simulink library "hcu_lib"  (R2021b)
settings: Solver=VariableStepAuto  StartTime=0.0  StopTime=10.0  RelTol=1e-3
undefined symbols (not defined in the file): ENUM_FAULTSTATE_FAIL, ENUM_FAULTSTATE_INDETERMINATE, ENUM_FAULTSTATE_PASS, EPSILON, FALSE, KPH2MPH, KPH2MPS, KXX2XX, MPH2KPH, MPS2KPH, ONE_INT, ONE_INT16, ONE_INT32, RADPS2RPM, RPM2RADPS, slcm, TRUE, UNDEFINED_VALUE, XX2KXX, ZERO_FLOAT, ZERO_INT, ZERO_INT16, ZERO_INT32
libraries: $bdroot x29, simulink x12, afl x1
(part 2 of 3)

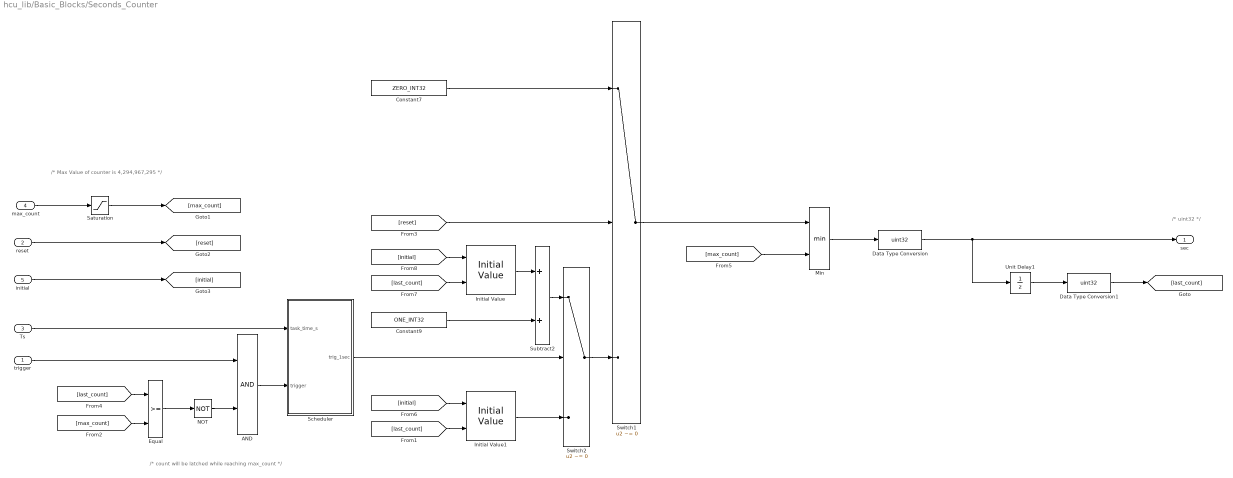
== system hcu_lib/Basic_Blocks/Seconds_Counter ==
  note: /* count will be latched while reaching max_count */
  note: /* uint32 */
  note: /* Max Value of counter is 4,294,967,295 */
  trigger : Inport
  reset : Inport  Port=2
  Ts : Inport  Port=3
  max_count : Inport  Port=4
  initial : Inport  Port=5
  AND : Logic  AllPortsSameDT=off  OutDataTypeStr=boolean
  Constant7 : Constant  Value=ZERO_INT32  OutDataTypeStr=uint16
  Constant9 : Constant  Value=ONE_INT32  OutDataTypeStr=single
  Data Type Conversion : DataTypeConversion  OutDataTypeStr=uint32
  Data Type Conversion1 : DataTypeConversion  OutDataTypeStr=uint32
  Equal : RelationalOperator  OutDataTypeStr=boolean  RndMeth=Simplest
  Initial Value : $bdroot/Basic_Blocks/Initial Value
  Initial Value1 : $bdroot/Basic_Blocks/Initial Value
  Min : MinMax  Inputs=2
  NOT : Logic  Operator=NOT  AllPortsSameDT=off  OutDataTypeStr=boolean
  Saturation : Saturate  UpperLimit=4294967295  LowerLimit=0
      settings: AttributesFormatString=<upper = %<UpperLimit>>\n<lower = %<LowerLimit>>
  Scheduler : Stateflow chart  TreatAsAtomicUnit=on
  Subtract2 : Sum
  Switch1 : Switch  Criteria=u2 ~= 0
      settings: AttributesFormatString=<%<Criteria>>
  Switch2 : Switch  Criteria=u2 ~= 0
      settings: AttributesFormatString=<%<Criteria>>
  Unit Delay1 : UnitDelay  SampleTime=-1  HasFrameUpgradeWarning=on
      settings: AttributesFormatString=<initial = %<X0>>
  sec : Outport
  wires:
  Data Type Conversion1/1 -> [last_count]
  Unit Delay1/1 -> Data Type Conversion1/1
  Data Type Conversion/1 -> Unit Delay1/1, sec/1
  Ts/1 -> Scheduler/1(task_time_s)
  Subtract2/1 -> Switch2/1
  Constant9/1 -> Subtract2/2
  Switch2/1 -> Switch1/3
  Constant7/1 -> Switch1/1
  max_count/1 -> Saturation/1
  Scheduler/1(trig_1sec) -> Switch2/2
  reset/1 -> [reset]
  [reset] -> Switch1/2
  Equal/1 -> NOT/1
  AND/1 -> Scheduler/2(trigger)
  trigger/1 -> AND/1
  NOT/1 -> AND/2
  [last_count] -> Equal/1
  Saturation/1 -> [max_count]
  [max_count] -> Equal/2
  [max_count] -> Min/2
  Min/1 -> Data Type Conversion/1
  Switch1/1 -> Min/1
  initial/1 -> [initial]
  Initial Value1/1 -> Switch2/3
  [last_count] -> Initial Value1/2
  [initial] -> Initial Value1/1
  Initial Value/1 -> Subtract2/1
  [initial] -> Initial Value/1
  [last_count] -> Initial Value/2

== system hcu_lib/Basic_Blocks/Test Detection Criteria ==
  trigger : Inport
  Ts : Inport  Port=2
  KDDM_xxxDTC_cnt : Inport  Port=3
  KDDM_xxxDetTO_s : Inport  Port=4
  Constant35 : Constant  Value=ZERO_INT
  Data Type Conversion : DataTypeConversion  OutDataTypeStr=single
  Data Type Conversion1 : DataTypeConversion  OutDataTypeStr=uint16
  Detect Increase : simulink/Logic and Bit Operations/Detect Increase  vinit=0.0  OutDataTypeStr=boolean
  Equal9 : RelationalOperator  Operator===  OutDataTypeStr=boolean  RndMeth=Simplest
  Gain : Gain  Gain=KXX2XX  RndMeth=Round
  Gain1 : Gain  Gain=KXX2XX
  Logical Operator19 : Logic  AllPortsSameDT=off  OutDataTypeStr=boolean
  Logical Operator3 : Logic  Operator=NOT  AllPortsSameDT=off  OutDataTypeStr=boolean
  ModMath : Subsystem  mask(Count){}
      mask help: Counter function.
      mask Display:
      | fprintf('ModMath');
      | port_label('output', 1, 'Remainder');
      | port_label('input', 1, 'Dividend');
      | port_label('input', 2, 'Divisor');
  Product : Product
  Rounding Function : Rounding  Operator=round
  Rounding Function1 : Rounding  Operator=round
  Timer : Subsystem  mask(Timer){}
      mask help: Timer funcion.
  VDDM_xxxDet_flg : Outport
  wires:
  Constant35/1 -> Equal9/2
  Logical Operator19/1 -> Detect Increase/1
  trigger/1 -> Timer/1(trigger), Logical Operator19/1, Logical Operator3/1
  [KDDM_xxxDetTO_s] -> Gain1/1
  Equal9/1 -> Logical Operator19/2
  Logical Operator3/1 -> Timer/2(reset)
  Timer/1(time) -> Gain/1
  Ts/1 -> Timer/3(Ts)
  Product/1 -> Timer/4(max_time)
  Data Type Conversion/1 -> Product/2
  KDDM_xxxDetTO_s/1 -> [KDDM_xxxDetTO_s], Product/1
  KDDM_xxxDTC_cnt/1 -> Data Type Conversion/1
  ModMath/1(Remainder) -> Data Type Conversion1/1
  Detect Increase/1 -> VDDM_xxxDet_flg/1
  Gain/1 -> Rounding Function/1
  Gain1/1 -> Rounding Function1/1
  Data Type Conversion1/1 -> Equal9/1
  Rounding Function/1 -> ModMath/1(Dividend)
  Rounding Function1/1 -> ModMath/2(Divisor)

== system hcu_lib/Basic_Blocks/Timer ==
  note: /* output signal type is single */
  trigger : Inport
  reset : Inport  Port=2
  Ts : Inport  Port=3
  max_time : Inport  Port=4
  Constant1 : Constant  Value=ZERO_FLOAT  OutDataTypeStr=single
  GreaterThan : RelationalOperator  Operator=<=  OutDataTypeStr=boolean  RndMeth=Simplest
  Subtract2 : Sum
  Switch : Switch  Criteria=u2 > Threshold
  Switch1 : Switch  Criteria=u2 ~= 0
      settings: AttributesFormatString=<%<Criteria>>
  Switch2 : Switch  Criteria=u2 ~= 0
      settings: AttributesFormatString=<%<Criteria>>
  Unit Delay1 : UnitDelay  SampleTime=-1  HasFrameUpgradeWarning=on
      settings: AttributesFormatString=<initial = %<X0>>
  time : Outport
  wires:
  [last_time] -> Subtract2/1
  max_time/1 -> Switch/1, GreaterThan/1
  Unit Delay1/1 -> [last_time], Switch1/3
  Switch/1 -> time/1, Unit Delay1/1
  Switch2/1 -> Switch/3, GreaterThan/2
  Ts/1 -> Subtract2/2
  Switch1/1 -> Switch2/3
  Constant1/1 -> Switch1/1
  reset/1 -> Switch1/2
  trigger/1 -> Switch2/2
  Subtract2/1 -> Switch2/1
  GreaterThan/1 -> Switch/2

== system hcu_lib/Basic_Blocks/derivative ==
  omega_radps : Inport
  task_time_s : Inport  Port=2
  Constant : Constant  Tag=struct('comment',struct('text','','placement',1),'output',struct('width',1,'name','$S_$B','unit','','type','Int16','offset',0,'max',NaN,'min',NaN,'freeze',1,'lsb',1,'arb',0,'class','default','address','','description','','value','0','tolerance',1,'show',0),'date',731450.689904282)  Value=0  OutDataTypeStr=single
  Constant1 : Constant  Tag=struct('comment',struct('text','','placement',1),'output',struct('width',1,'name','$S_$B','unit','','type','Int16','offset',0,'max',NaN,'min',NaN,'freeze',1,'lsb',1,'arb',0,'class','default','address','','description','','value','2','tolerance',1,'show',0),'date',731450.690075)  Value=TRUE
  Product : Product  Tag=struct('comment',struct('text','','placement',1),'logdata',struct('maxnumvals',inf,'plotchannels',[],'stepsize',0,'downsampling',1,'loggingmode',3,'channels',1),'output',struct('width',1,'name','$S_$B','unit','','type','Int32Bin15','offset',0,'max',65535,'min',-65536,'freeze',1,'lsb',2^-15,'arb',0,'class','default','address','','description','','autoscalingmode',1,'lowerheadroom',1,'upperheadroom',1,'headroomunit','bit','checkmin',0,'checkmax',0,'show',0),'inputs','*/','exceptionhandling',1,'date',731458.438505301)  Inputs=*/  InputSameDT=on  RndMeth=Zero  SaturateOnIntegerOverflow=on  OutDataTypeStr=Inherit: Same as first input
  Saturation1 : Saturate  Tag=struct('comment',struct('text','','placement',1),'logdata',struct('maxnumvals',inf,'plotchannels',[],'stepsize',0,'downsampling',1,'loggingmode',3,'channels',1),'output',struct('width',1,'name','$S_$B','unit','s','type','Time16bin10','offset',0,'max',63.999,'min',0,'freeze',1,'lsb',2^-10,'arb',0,'class','default','address','','description','','autoscalingmode',1,'lowerheadroom',1,'upperheadroom',1,'headroomunit','bit','show',0),'lowerlimit',struct('width',1,'name','$S_$B_lower','unit','','type','Int16','offset',0,'max',NaN,'min',NaN,'freeze',1,'lsb',1,'arb',0,'class','default','address','','description','','value','12e-3','scalar',0),'upperlimit',struct('width',1,'name','$S_$B_upper','unit','','type','Int16','offset',0,'max',NaN,'min',NaN,'freeze',1,'lsb',1,'arb',0,'class','default','address','','description','','value','63.9','scalar',0),'date',731458.439118333)  UpperLimit=63.9  LowerLimit=12e-3
  Saturation2 : Saturate  Tag=struct('comment',struct('text','','placement',1),'logdata',struct('maxnumvals',inf,'plotchannels',[],'stepsize',0,'downsampling',1,'loggingmode',3,'channels',1),'output',struct('width',1,'name','$S_$B','unit','','type','Int32Bin15','offset',0,'max',65535,'min',-65536,'freeze',1,'lsb',2^-15,'arb',0,'class','default','address','','description','','autoscalingmode',1,'lowerheadroom',1,'upperheadroom',1,'headroomunit','bit','show',0),'lowerlimit',struct('width',1,'name','$S_$B_lower','unit','','type','Int16','offset',0,'max',NaN,'min',NaN,'freeze',1,'lsb',1,'arb',0,'class','default','address','','description','','value','-65536','scalar',0),'upperlimit',struct('width',1,'name','$S_$B_upper','unit','','type','Int16','offset',0,'max',NaN,'min',NaN,'freeze',1,'lsb',1,'arb',0,'class','default','address','','description','','value','65535','scalar',0),'date',731455.58891853)  UpperLimit=65535  LowerLimit=-65536
  Sum : Sum  Tag=struct('comment',struct('text','','placement',1),'logdata',struct('maxnumvals',inf,'plotchannels',[],'stepsize',0,'downsampling',1,'loggingmode',3,'channels',1),'output',struct('width',1,'name','$S_$B','unit','','type','Int32Bin15','offset',0,'max',65535,'min',-65536,'freeze',1,'lsb',2^-15,'arb',0,'class','default','address','','description','','autoscalingmode',1,'lowerheadroom',1,'upperheadroom',1,'headroomunit','bit','checkmin',0,'checkmax',0,'show',0),'inputs','+-','date',731450.688943275)  Inputs=+-  InputSameDT=on  SaturateOnIntegerOverflow=on  OutDataTypeStr=Inherit: Same as first input
  Switch : Switch  Tag=struct('comment',struct('text','','placement',1),'logdata',struct('maxnumvals',inf,'plotchannels',[],'stepsize',0,'downsampling',1,'loggingmode',3,'channels',1),'output',struct('width',1,'name','$S_$B','unit','','type','Int32Bin15','offset',0,'max',65535,'min',-65536,'freeze',1,'lsb',2^-15,'arb',0,'class','default','address','','description','','autoscalingmode',1,'lowerheadroom',1,'upperheadroom',1,'headroomunit','bit','checkmin',0,'checkmax',0,'show',0),'threshold',struct('width',1,'name','$S_$B_threshold','unit','','type','Int16','offset',0,'max',NaN,'min',NaN,'freeze',1,'lsb',1,'arb',0,'class','default','address','','description','','value','1','scalar',0),'date',731458.438569977)  Threshold=0.5  SaturateOnIntegerOverflow=on  InputSameDT=on
  UnitDelay1 : UnitDelay  Tag=struct('comment',struct('text','','placement',1),'logdata',struct('maxnumvals',inf,'plotchannels',[],'stepsize',0,'downsampling',1,'loggingmode',3,'channels',1),'output',struct('width',1,'name','$S_$B','unit','','type','Int32Bin15','offset',0,'max',65535,'min',-65536,'freeze',1,'lsb',2^-15,'arb',0,'class','default','address','','description','','autoscalingmode',1,'lowerheadroom',1,'upperheadroom',1,'headroomunit','bit','checkmin',0,'checkmax',0,'show',0,'initial','0'),'state',0,'dt','-1','date',731450.687911019)  SampleTime=-1  HasFrameUpgradeWarning=on
  UnitDelay2 : UnitDelay  Tag=struct('comment',struct('text','','placement',1),'logdata',struct('maxnumvals',inf,'plotchannels',[],'stepsize',0,'downsampling',1,'loggingmode',3,'channels',1),'output',struct('width',1,'name','$S_$B','unit','','type','UInt8','offset',0,'max',255,'min',0,'freeze',1,'lsb',1,'arb',0,'class','default','address','','description','','autoscalingmode',1,'lowerheadroom',1,'upperheadroom',1,'headroomunit','bit','checkmin',0,'checkmax',0,'show',0,'initial','0'),'state',0,'dt','-1','date',731450.690382801)  InitialCondition=FALSE  SampleTime=-1  StateName=first_pass  HasFrameUpgradeWarning=on
  rot_acc_radps2 : Outport
  wires:
  Saturation1/1 -> Product/2
  Constant1/1 -> UnitDelay2/1
  UnitDelay2/1 -> Switch/2
  Constant/1 -> Switch/3  "zero"
  Switch/1 -> Product/1
  task_time_s/1 -> Saturation1/1
  Sum/1 -> Switch/1
  Product/1 -> Saturation2/1
  UnitDelay1/1 -> Sum/2
  Saturation2/1 -> rot_acc_radps2/1  "rot_acc_radps2"
  omega_radps/1 -> Sum/1, UnitDelay1/1

== system hcu_lib/Basic_Blocks/divide ==
  dividend : Inport
  divisor : Inport  Port=2
  default_value : Inport  Port=3
  Divide : Product  Inputs=*/
  Interval Test : simulink/Logic and Bit Operations/Interval Test  IntervalClosedRight=on  uplimit=single(0.00001)  IntervalClosedLeft=on  lowlimit=single(-0.00001)  OutDataTypeStr=boolean
  Logical Operator : Logic  Operator=NOT  Inputs=1  AllPortsSameDT=off  OutDataTypeStr=boolean
  Switch : Switch  Threshold=0.5
  quotient : Outport
  wires:
  Logical Operator/1 -> Switch/2
  default_value/1 -> Switch/3  "default_value"
  Interval Test/1 -> Logical Operator/1
  Switch/1 -> quotient/1
  Divide/1 -> Switch/1
  divisor/1 -> Interval Test/1, Divide/2  "divisor"
  dividend/1 -> Divide/1  "dividend"

== system hcu_lib/Basic_Blocks/rolling average ==
  note: new_average = [ (sample_interval)/(sample_interval + time_constant) ] * (new_value - old_ave) + old_ave
  note: - (FK_TMR/TC)
      |                                    f  =  1  -  e
      |
      |       Where "f" is called the filter constant in the difference equation:
      |
      |                    new_average = f * new_value + (1 - f) * old_average
  note: Using the first two terms of the series expansion:
      |
      |                     x                     x2
      |                                e   =  1  +  x  +  --  + ......
      |                                           2!
      |
      |       Simplifying, the exponential "f" becomes:
      |
      |                  - (FK_TMR/TC)              1
      |           f  =  1  -  e                    =  1  -  -------------  =  . . .
      |                                                    (FK_TMR/TC)
      |                           e
      |
      |                              1                      1
      |          f  =  1  -  ---------------------------------  =    ------------------- .
      |                                  1 + (FK_TMR / TC)       1 + (TC / FK_TMR)
  new_value : Inport
  old_ave : Inport  Port=2
  delta_t : Inport  Port=3
  tc : Inport  Port=4
  IC : UnitDelay  Tag=struct('comment',struct('text','','placement',1),'logdata',struct('maxnumvals',inf,'plotchannels',[],'stepsize',0,'downsampling',1,'loggingmode',3,'channels',1),'output',struct('width',1,'name','$S_$B','unit','','type','Int16','offset',0,'max',NaN,'min',NaN,'freeze',1,'lsb',1,'arb',0,'class','default','address','','description','','autoscalingmode',1,'lowerheadroom',1,'upperheadroom',1,'headroomunit','bit','checkmin',0,'checkmax',0,'show',0,'initial','2'),'state',0,'dt','-1','date',731455.586925799)  InitialCondition=1  SampleTime=-1  HasFrameUpgradeWarning=on
  Product_tmp1 : Product  Tag=struct('comment',struct('text','','placement',1),'logdata',struct('maxnumvals',inf,'plotchannels',[],'stepsize',0,'downsampling',1,'loggingmode',3,'channels',1),'output',struct('width',1,'name','$S_$B','unit','','type','Int32Bin15','offset',0,'max',65535,'min',-65536,'freeze',1,'lsb',2^-15,'arb',0,'class','default','address','','description','','autoscalingmode',1,'lowerheadroom',1,'upperheadroom',1,'headroomunit','bit','checkmin',0,'checkmax',0,'show',0),'inputs','**','exceptionhandling',1,'date',731455.58640515)  Inputs=**  InputSameDT=on  RndMeth=Zero  OutDataTypeStr=Inherit: Same as first input
  Sum : Sum  Tag=struct('comment',struct('text','','placement',1),'logdata',struct('maxnumvals',inf,'plotchannels',[],'stepsize',0,'downsampling',1,'loggingmode',3,'channels',1),'output',struct('width',1,'name','$S_$B','unit','','type','Int32Bin15','offset',0,'max',65535,'min',-65536,'freeze',1,'lsb',2^-15,'arb',0,'class','default','address','','description','','autoscalingmode',1,'lowerheadroom',1,'upperheadroom',1,'headroomunit','bit','checkmin',0,'checkmax',0,'show',0),'inputs','-+','date',731455.586330463)  Inputs=-+  InputSameDT=on  OutDataTypeStr=Inherit: Same as first input
  Sum1 : Sum  Tag=struct('comment',struct('text','','placement',1),'logdata',struct('maxnumvals',inf,'plotchannels',[],'stepsize',0,'downsampling',1,'loggingmode',3,'channels',1),'output',struct('width',1,'name','$S_$B','unit','','type','Int32Bin15','offset',0,'max',65535,'min',-65536,'freeze',1,'lsb',2^-15,'arb',0,'class','default','address','','description','','autoscalingmode',1,'lowerheadroom',1,'upperheadroom',1,'headroomunit','bit','checkmin',0,'checkmax',0,'show',0),'inputs','++','date',731455.58628235)  InputSameDT=on  OutDataTypeStr=Inherit: Same as first input
  Sum2 : Sum  Tag=struct('comment',struct('text','','placement',1),'logdata',struct('maxnumvals',inf,'plotchannels',[],'stepsize',0,'downsampling',1,'loggingmode',3,'channels',1),'output',struct('width',1,'name','$S_$B','unit','','type','Int32Bin15','offset',0,'max',65535,'min',-65536,'freeze',1,'lsb',2^-15,'arb',0,'class','default','address','','description','','autoscalingmode',1,'lowerheadroom',1,'upperheadroom',1,'headroomunit','bit','checkmin',0,'checkmax',0,'show',0),'inputs','++','date',731455.586506424)  InputSameDT=on  OutDataTypeStr=Inherit: Same as first input
  Switch1 : Switch  Tag=struct('comment',struct('text','','placement',1),'logdata',struct('maxnumvals',inf,'plotchannels',[],'stepsize',0,'downsampling',1,'loggingmode',3,'channels',1),'output',struct('width',1,'name','$S_$B','unit','','type','Int32Bin15','offset',0,'max',65535,'min',-65536,'freeze',1,'lsb',2^-15,'arb',0,'class','default','address','','description','','autoscalingmode',1,'lowerheadroom',1,'upperheadroom',1,'headroomunit','bit','checkmin',0,'checkmax',0,'show',0),'threshold',struct('width',1,'name','$S_$B_threshold','unit','','type','Int16','offset',0,'max',NaN,'min',NaN,'freeze',1,'lsb',1,'arb',0,'class','default','address','','description','','value','1','scalar',0),'date',731455.58657044)  Threshold=0.5  InputSameDT=on
  divide : $bdroot/Basic_Blocks/divide
  zero : Constant  Tag=struct('comment',struct('text','','placement',1),'output',struct('width',1,'name','$S_$B','unit','','type','Int16','offset',0,'max',NaN,'min',NaN,'freeze',1,'lsb',1,'arb',0,'class','default','address','','description','','value','0','tolerance',1,'show',0),'date',731455.58675544)  Value=0  OutDataTypeStr=Inherit: Inherit via back propagation
  zero1 : Constant  Tag=struct('comment',struct('text','','placement',1),'output',struct('width',1,'name','$S_$B','unit','','type','Int16','offset',0,'max',NaN,'min',NaN,'freeze',1,'lsb',1,'arb',0,'class','default','address','','description','','value','0','tolerance',1,'show',0),'date',731455.58675544)  Value=0  OutDataTypeStr=Inherit: Inherit via back propagation
  new_ave : Outport
  wires:
  zero1/1 -> divide/3
  Product_tmp1/1 -> divide/1
  [new_value] -> Switch1/1
  Switch1/1 -> new_ave/1  "new_ave"
  Sum2/1 -> Switch1/3  "new_ave"
  IC/1 -> Switch1/2
  zero/1 -> IC/1
  Sum1/1 -> divide/2
  Sum/1 -> Product_tmp1/1
  divide/1 -> Sum2/2
  tc/1 -> Sum1/2
  delta_t/1 -> Sum1/1, Product_tmp1/2  "delta_t"
  new_value/1 -> [new_value]  "new_value"
  old_ave/1 -> Sum2/1, Sum/1  "old_ave"
  [new_value] -> Sum/2

== system hcu_lib/IO_Signal_Process_Blocks/CAN_Msg_Validity_Process ==
  signal_in : Inport
  inverse_flag : Inport  Port=2
  debounce_sat : Inport  Port=3
  debounce_inc : Inport  Port=4
  debounce_dec : Inport  Port=5
  cal_override_flag : Inport  Port=6
  cal_override_value : Inport  Port=7
  service_flag : Inport  Port=8
  service_value : Inport  Port=9
  AFL : afl/AFL  SystemSampleTime=-1
  Ground : Ground
  Ground1 : Ground
  Ground2 : Ground
  Logical Operator : Logic  Operator=NOT  Inputs=1  AllPortsSameDT=off  OutDataTypeStr=boolean
  SRS_HCU_INP_003 : simulink/Model-Wide Utilities/DocBlock  DocumentType=Text
  Switch1 : Switch  Criteria=u2 ~= 0  Threshold=0.5
  Terminator : Terminator
  Terminator1 : Terminator
  Terminator2 : Terminator
  "override_signal_m2 " : $bdroot/Signal_Process_Blocks/override_signal_m2 
  signal_out : Outport  OutDataTypeStr=boolean
  wires:
  "override_signal_m2 "/1 -> signal_out/1
  AFL/3 -> Terminator/1
  "override_signal_m2 "/2 -> Terminator1/1
  AFL/1 -> "override_signal_m2 "/2
  Ground/1 -> "override_signal_m2 "/1
  service_flag/1 -> "override_signal_m2 "/3
  service_value/1 -> "override_signal_m2 "/4
  cal_override_flag/1 -> "override_signal_m2 "/5
  cal_override_value/1 -> "override_signal_m2 "/6
  inverse_flag/1 -> Switch1/2
  signal_in/1 -> Switch1/3, Logical Operator/1
  Switch1/1 -> AFL/1
  Logical Operator/1 -> Switch1/1
  AFL/2 -> Terminator2/1
  debounce_sat/1 -> AFL/2
  debounce_inc/1 -> AFL/3
  debounce_dec/1 -> AFL/4
  Ground1/1 -> AFL/5
  Ground2/1 -> AFL/6

== system hcu_lib/IO_Signal_Process_Blocks/Protect ==
  in : Inport
  Bias : Bias  Bias=1
  Bitwise Operator : simulink/Logic and Bit Operations/Bitwise Operator  logicop=NOT  UseBitMask=off  BitMask=bin2dec('11011001')  BitMaskRealWorld=Stored Integer
  out : Outport
  wires:
  Bitwise Operator/1 -> Bias/1
  Bias/1 -> out/1
  in/1 -> Bitwise Operator/1

== system hcu_lib/IO_Signal_Process_Blocks/RollCnt ==
  max : Inport
  Add : Sum
  Constant : Constant  OutDataTypeStr=Inherit: Inherit via back propagation
  Constant1 : Constant  Value=0  OutDataTypeStr=Inherit: Inherit via back propagation
  Data Type Conversion6 : DataTypeConversion  OutDataTypeStr=uint8
  Relational Operator : RelationalOperator  Operator=>  OutDataTypeStr=boolean  RndMeth=Nearest
  Switch2 : Switch  Criteria=u2 ~= 0
  Unit Delay1 : UnitDelay  SampleTime=-1  HasFrameUpgradeWarning=on
      settings: AttributesFormatString=<initial=%<X0>>
  out : Outport
  wires:
  Constant/1 -> Add/1
  Add/1 -> Switch2/3, Relational Operator/1
  Unit Delay1/1 -> Add/2
  Constant1/1 -> Switch2/1
  Switch2/1 -> Unit Delay1/1, Data Type Conversion6/1
  max/1 -> Relational Operator/2
  Relational Operator/1 -> Switch2/2
  Data Type Conversion6/1 -> out/1

== system hcu_lib/IO_Signal_Process_Blocks/RollCntValid ==
  RollCnt : Inport
  TimeOut : Inport  Port=2
  Ts : Inport  Port=3
  Add : Sum
  RESET : Constant  Value=0  OutDataTypeStr=single
  Relational Operator1 : RelationalOperator  Operator===  OutDataTypeStr=boolean  RndMeth=Nearest
  Relational Operator2 : RelationalOperator  Operator=<  OutDataTypeStr=boolean  RndMeth=Nearest
  Switch : Switch  Criteria=u2 ~= 0
  Unit Delay : UnitDelay  SampleTime=-1  HasFrameUpgradeWarning=on
  Unit Delay1 : UnitDelay  SampleTime=-1  HasFrameUpgradeWarning=on
  valid : Outport
  wires:
  Ts/1 -> Add/2
  Add/1 -> Switch/1
  Unit Delay/1 -> Add/1
  RollCnt/1 -> Unit Delay1/1, Relational Operator1/2
  Unit Delay1/1 -> Relational Operator1/1
  Switch/1 -> Unit Delay/1, Relational Operator2/1
  Relational Operator1/1 -> Switch/2
  RESET/1 -> Switch/3
  TimeOut/1 -> Relational Operator2/2
  Relational Operator2/1 -> valid/1

== system hcu_lib/IO_Signal_Process_Blocks/can_signal_process ==
  signal_in : Inport
  signal_valid_in : Inport  Port=2
  msg_valid : Inport  Port=3
  default_value : Inport  Port=4
  fault_filter_lim : Inport  Port=5
  fault_filter_inc : Inport  Port=6
  fault_filter_dec : Inport  Port=7
  invalid_override : Inport  Port=8
  valid_override : Inport  Port=9
  cal_ovrdflg : Inport  Port=10
  cal_ovrdval : Inport  Port=11
  service_flag : Inport  Port=12
  service_value : Inport  Port=13
  Logical Operator1 : Logic  Operator=NOT  AllPortsSameDT=off  OutDataTypeStr=boolean
  Logical Operator2 : Logic  AllPortsSameDT=off  OutDataTypeStr=boolean
  "override_signal_m2 " : $bdroot/Signal_Process_Blocks/override_signal_m2 
  sig_valid_check : $bdroot/Signal_Process_Blocks/sig_valid_check
  signal_out : Outport
  signal_valid_out : Outport  Port=2
  wires:
  "override_signal_m2 "/2 -> signal_valid_out/1
  "override_signal_m2 "/1 -> signal_out/1
  msg_valid/1 -> Logical Operator2/2
  signal_in/1 -> sig_valid_check/1
  signal_valid_in/1 -> Logical Operator2/1
  Logical Operator2/1 -> sig_valid_check/2
  invalid_override/1 -> sig_valid_check/3
  Logical Operator1/1 -> "override_signal_m2 "/1  "signal_valid_flg_raw"
  service_flag/1 -> "override_signal_m2 "/3
  service_value/1 -> "override_signal_m2 "/4
  cal_ovrdflg/1 -> "override_signal_m2 "/5
  cal_ovrdval/1 -> "override_signal_m2 "/6
  valid_override/1 -> sig_valid_check/4
  default_value/1 -> sig_valid_check/5
  fault_filter_lim/1 -> sig_valid_check/6
  fault_filter_inc/1 -> sig_valid_check/7
  fault_filter_dec/1 -> sig_valid_check/8
  sig_valid_check/1 -> Logical Operator1/1  "fault_flg"
  sig_valid_check/2 -> "override_signal_m2 "/2  "valid_flg"

== system hcu_lib/IO_Signal_Process_Blocks/digital_signal_process ==
  signal_in : Inport
  inverse_flag : Inport  Port=2
  debounce_sat : Inport  Port=3
  debounce_inc : Inport  Port=4
  debounce_dec : Inport  Port=5
  cal_override_flag : Inport  Port=6
  cal_override_value : Inport  Port=7
  service_flag : Inport  Port=8
  service_value : Inport  Port=9
  Ground : Ground
  Logical Operator : Logic  Operator=NOT  Inputs=1  AllPortsSameDT=off  OutDataTypeStr=boolean
  Switch1 : Switch  Criteria=u2 ~= 0  Threshold=0.5
  Terminator : Terminator
  Terminator1 : Terminator
  fault_filter_reset : Subsystem  AncestorBlock=hcu_lib/Signal_Process_Blocks/fault_filter_reset  TreatAsAtomicUnit=on  RTWFcnName=ff_reset  RTWFileName=HCU_LIB  mask(FaultFilterReset){}
      mask help: Fault filter reset.
      settings: RTWFcnNameOpts=Use subsystem name  RTWFileNameOpts=User specified
  "override_signal_m2 " : $bdroot/Signal_Process_Blocks/override_signal_m2 
  signal_out : Outport  OutDataTypeStr=boolean
  wires:
  debounce_dec/1 -> fault_filter_reset/4(dec)
  debounce_inc/1 -> fault_filter_reset/3(inc)
  debounce_sat/1 -> fault_filter_reset/2(sat)
  "override_signal_m2 "/1 -> signal_out/1
  fault_filter_reset/2(ff_count) -> Terminator/1
  "override_signal_m2 "/2 -> Terminator1/1
  fault_filter_reset/1(fault_flg) -> "override_signal_m2 "/2
  Ground/1 -> "override_signal_m2 "/1
  service_flag/1 -> "override_signal_m2 "/3
  service_value/1 -> "override_signal_m2 "/4
  cal_override_flag/1 -> "override_signal_m2 "/5
  cal_override_value/1 -> "override_signal_m2 "/6
  inverse_flag/1 -> Switch1/2
  signal_in/1 -> Switch1/3, Logical Operator/1
  Switch1/1 -> fault_filter_reset/1(i_deb)
  Logical Operator/1 -> Switch1/1

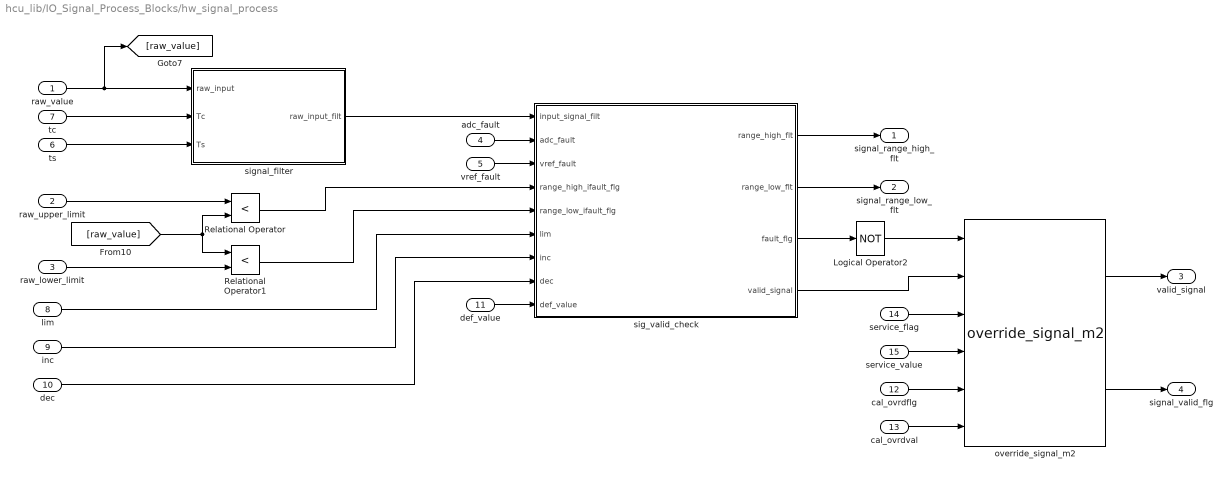
== system hcu_lib/IO_Signal_Process_Blocks/hw_signal_process ==
  raw_value : Inport
  raw_upper_limit : Inport  Port=2
  raw_lower_limit : Inport  Port=3
  adc_fault : Inport  Port=4
  vref_fault : Inport  Port=5
  ts : Inport  Port=6
  tc : Inport  Port=7
  lim : Inport  Port=8
  inc : Inport  Port=9
  dec : Inport  Port=10
  def_value : Inport  Port=11
  cal_ovrdflg : Inport  Port=12
  cal_ovrdval : Inport  Port=13
  service_flag : Inport  Port=14
  service_value : Inport  Port=15
  Logical Operator2 : Logic  Operator=NOT  AllPortsSameDT=off  OutDataTypeStr=boolean
  Relational Operator : RelationalOperator  Operator=<  OutDataTypeStr=boolean  RndMeth=Nearest
  Relational Operator1 : RelationalOperator  Operator=<  OutDataTypeStr=boolean  RndMeth=Nearest
  "override_signal_m2 " : $bdroot/Signal_Process_Blocks/override_signal_m2 
  sig_valid_check : Subsystem  RTWFcnName=sig_valid_check
      settings: RTWFcnNameOpts=User specified
  signal_filter : Subsystem
  signal_range_high_flt : Outport
  signal_range_low_flt : Outport  Port=2
  valid_signal : Outport  Port=3
  signal_valid_flg : Outport  Port=4
  wires:
  Logical Operator2/1 -> "override_signal_m2 "/1
  ts/1 -> signal_filter/3(Ts)
  tc/1 -> signal_filter/2(Tc)
  raw_value/1 -> [raw_value], signal_filter/1(raw_input)
  Relational Operator/1 -> sig_valid_check/4(range_high_ifault_flg)
  [raw_value] -> Relational Operator1/1, Relational Operator/2
  def_value/1 -> sig_valid_check/9(def_value)
  dec/1 -> sig_valid_check/8(dec)
  inc/1 -> sig_valid_check/7(inc)
  lim/1 -> sig_valid_check/6(lim)
  raw_lower_limit/1 -> Relational Operator1/2
  raw_upper_limit/1 -> Relational Operator/1
  sig_valid_check/3(fault_flg) -> Logical Operator2/1
  signal_filter/1(raw_input_filt) -> sig_valid_check/1(input_signal_filt)
  Relational Operator1/1 -> sig_valid_check/5(range_low_ifault_flg)
  sig_valid_check/1(range_high_flt) -> signal_range_high_flt/1
  sig_valid_check/2(range_low_flt) -> signal_range_low_flt/1
  service_flag/1 -> "override_signal_m2 "/3
  service_value/1 -> "override_signal_m2 "/4
  cal_ovrdflg/1 -> "override_signal_m2 "/5
  cal_ovrdval/1 -> "override_signal_m2 "/6
  sig_valid_check/4(valid_signal) -> "override_signal_m2 "/2
  "override_signal_m2 "/1 -> valid_signal/1
  "override_signal_m2 "/2 -> signal_valid_flg/1
  adc_fault/1 -> sig_valid_check/2(adc_fault)
  vref_fault/1 -> sig_valid_check/3(vref_fault)

== system hcu_lib/IO_Signal_Process_Blocks/signal_out ==
  in : Inport
  srvcflg : Inport  Port=2
  srvcval : Inport  Port=3
  ovrdflg : Inport  Port=4
  ovrdval : Inport  Port=5
  Constant1 : Constant  Value=TRUE  OutDataTypeStr=Inherit: Inherit via back propagation
  Terminator13 : Terminator
  "override_signal_m2 " : $bdroot/Signal_Process_Blocks/override_signal_m2 
  out : Outport
  wires:
  in/1 -> "override_signal_m2 "/2
  "override_signal_m2 "/1 -> out/1
  Constant1/1 -> "override_signal_m2 "/1
  srvcflg/1 -> "override_signal_m2 "/3
  srvcval/1 -> "override_signal_m2 "/4
  ovrdflg/1 -> "override_signal_m2 "/5
  ovrdval/1 -> "override_signal_m2 "/6
  "override_signal_m2 "/2 -> Terminator13/1

== system hcu_lib/Model Info1/EmptySubsystem ==

== system hcu_lib/Signal_Conversion_Blocks/Raw32 ==
  input : Inport
  gain : Inport  Port=2
  offset : Inport  Port=3
  Add1 : Sum  Inputs=+-
  Constant : Constant  Value=EPSILON
  Data Type Conversion6 : DataTypeConversion  OutDataTypeStr=uint32
  Divide : Product  Inputs=*/
  MinMax : MinMax  Function=max  Inputs=2
  Rounding Function : Rounding  Operator=round
  raw_value : Outport
  wires:
  Data Type Conversion6/1 -> raw_value/1
  Rounding Function/1 -> Data Type Conversion6/1
  input/1 -> Add1/1
  offset/1 -> Add1/2
  Add1/1 -> Divide/1
  Divide/1 -> Rounding Function/1
  gain/1 -> MinMax/1
  MinMax/1 -> Divide/2
  Constant/1 -> MinMax/2

== system hcu_lib/Signal_Conversion_Blocks/conv_counts_to_eng_units ==
  signal : Inport
  gain : Inport  Port=2
  offset : Inport  Port=3
  Product : Product  RndMeth=Zero
  Sum : Sum
  output_signal : Outport
  wires:
  Product/1 -> Sum/1
  gain/1 -> Product/1  "gain"
  signal/1 -> Product/2  "signal"
  offset/1 -> Sum/2  "offset"
  Sum/1 -> output_signal/1  "output_signal"

== system hcu_lib/Signal_Conversion_Blocks/conv_eng_units_to_counts ==
  input : Inport
  gain : Inport  Port=2
  offset : Inport  Port=3
  Constant : Constant  Value=0  OutDataTypeStr=Inherit: Inherit via back propagation
  Sum : Sum  Inputs=+-
  divide : $bdroot/Basic_Blocks/divide
  output_signal : Outport
  wires:
  Constant/1 -> divide/3
  offset/1 -> Sum/2  "offset"
  input/1 -> Sum/1  "input"
  gain/1 -> divide/2  "gain"
  Sum/1 -> divide/1  "out_signal"
  divide/1 -> output_signal/1  "output_signal"

== system hcu_lib/Signal_Conversion_Blocks/convert_in ==
  raw32 : Inport
  Add : Sum
  Data Type Conversion : DataTypeConversion  OutDataTypeStr=single
  Product : Product  RndMeth=Zero
  gain : Constant  Value=single(gain)  OutDataTypeStr=single
  offset : Constant  Value=single(offset)  OutDataTypeStr=single
  value : Outport
  wires:
  raw32/1 -> Data Type Conversion/1
  gain/1 -> Product/2
  Product/1 -> Add/1
  offset/1 -> Add/2
  Add/1 -> value/1
  Data Type Conversion/1 -> Product/1

== system hcu_lib/Signal_Conversion_Blocks/convert_out ==
  value : Inport
  Add : Sum  Inputs=+-
  Constant : Constant  Value=EPSILON
  Data Type Conversion : DataTypeConversion  OutDataTypeStr=uint32  RndMeth=Nearest
  Divide : Product  Inputs=*/
  MinMax : MinMax  Function=max  Inputs=2
  gain : Constant  Value=single(gain)  OutDataTypeStr=single
  offset : Constant  Value=single(offset)  OutDataTypeStr=single
  raw32 : Outport
  wires:
  value/1 -> Add/1
  offset/1 -> Add/2
  Divide/1 -> Data Type Conversion/1
  Add/1 -> Divide/1
  Data Type Conversion/1 -> raw32/1
  gain/1 -> MinMax/1
  Constant/1 -> MinMax/2
  MinMax/1 -> Divide/2

== system hcu_lib/Signal_Process_Blocks/fault_filter_latch ==
  i_fault : Inport
  sat : Inport  Port=2
  inc : Inport  Port=3
  dec : Inport  Port=4
  Add : Sum
  Constant : Constant  Value=0  OutDataTypeStr=Inherit: Inherit via back propagation
  Gain : Gain  Gain=-1
  MinMax : MinMax  Inputs=2
  MinMax1 : MinMax  Function=max  Inputs=2
  Relational Operator : RelationalOperator  OutDataTypeStr=boolean  RndMeth=Nearest
  Switch : Switch
  Switch1 : Switch
  Unit Delay : UnitDelay  SampleTime=-1  HasFrameUpgradeWarning=on
  Unit Delay1 : UnitDelay  SampleTime=-1  HasFrameUpgradeWarning=on
  fault_flg : Outport
  ff_count : Outport  Port=2
  wires:
  inc/1 -> Switch/1  "inc"
  dec/1 -> Gain/1  "dec"
  i_fault/1 -> Switch/2  "i_fault"
  Switch/1 -> Add/1
  Unit Delay/1 -> Add/2
  Gain/1 -> Switch/3
  Add/1 -> MinMax/1
  Constant/1 -> MinMax/2
  MinMax/1 -> MinMax1/1
  MinMax1/1 -> ff_count/1, Unit Delay/1, Relational Operator/1
  sat/1 -> MinMax1/2, Relational Operator/2  "sat"
  Relational Operator/1 -> Switch1/2, Switch1/1
  Switch1/1 -> fault_flg/1, Unit Delay1/1
  Unit Delay1/1 -> Switch1/3

== system hcu_lib/Signal_Process_Blocks/fault_filter_reset ==
  i_fault : Inport
  sat : Inport  Port=2
  inc : Inport  Port=3
  dec : Inport  Port=4
  Add : Sum
  Add1 : Sum  Inputs=+-
  Constant : Constant  Value=0  OutDataTypeStr=uint8
  Data Type Conversion : DataTypeConversion  OutDataTypeStr=int16
  MinMax : MinMax  Function=max  Inputs=2
  MinMax1 : MinMax  Inputs=2
  Relational Operator : RelationalOperator  OutDataTypeStr=boolean  RndMeth=Nearest
  Switch : Switch  Criteria=u2 ~= 0
  Unit Delay : UnitDelay  SampleTime=-1  HasFrameUpgradeWarning=on
  fault_flg : Outport
  ff_count : Outport  Port=2
  wires:
  inc/1 -> Add/2  "inc"
  dec/1 -> Add1/2  "dec"
  i_fault/1 -> Switch/2  "i_fault"
  Unit Delay/1 -> Add/1, Add1/1
  Constant/1 -> MinMax/2
  MinMax/1 -> MinMax1/1
  MinMax1/1 -> ff_count/1, Unit Delay/1, Relational Operator/1
  sat/1 -> MinMax1/2, Relational Operator/2  "sat"
  Relational Operator/1 -> fault_flg/1
  Add/1 -> Switch/1
  Add1/1 -> Switch/3
  Switch/1 -> Data Type Conversion/1
  Data Type Conversion/1 -> MinMax/1

== system hcu_lib/Signal_Process_Blocks/latching fault filter reinit ==
  i_fault : Inport
  sat : Inport  Port=2
  inc : Inport  Port=3
  dec : Inport  Port=4
  reinit : Inport  Port=5
  lff_ctl : Stateflow chart  TreatAsAtomicUnit=on
  fault_flg : Outport
  ff_count : Outport  Port=2
  wires:
  reinit/1 -> lff_ctl/5(reinit)  "reinit"
  lff_ctl/2(ff_count) -> ff_count/1  "ff_count"
  sat/1 -> lff_ctl/1(sat)  "sat"
  inc/1 -> lff_ctl/2(inc)  "inc"
  lff_ctl/1(fault_flg) -> fault_flg/1  "fault_flg"
  i_fault/1 -> lff_ctl/4(i_fault)  "i_fault"
  dec/1 -> lff_ctl/3(dec)  "dec"

== system hcu_lib/Signal_Process_Blocks/latching_fault_filter ==
  i_fault : Inport
  sat : Inport  Port=2
  inc : Inport  Port=3
  dec : Inport  Port=4
  lff_ctl : Stateflow chart  TreatAsAtomicUnit=on
  fault_flg : Outport
  ff_count : Outport  Port=2
  wires:
  dec/1 -> lff_ctl/3(dec)  "dec"
  i_fault/1 -> lff_ctl/4(i_fault)  "i_fault"
  lff_ctl/1(fault_flg) -> fault_flg/1  "fault_flg"
  inc/1 -> lff_ctl/2(inc)  "inc"
  sat/1 -> lff_ctl/1(sat)  "sat"
  lff_ctl/2(ff_count) -> ff_count/1  "ff_count"

== system hcu_lib/Signal_Process_Blocks/override_signal_m1 ==
  note: When either service_ovrdflg or cal_ovrdflg is true, signal_valid_flg is set as TRUE
  note: ONLY ONE ovrdflg (Service_ovrdflg and Cal_ovrdflg) can be valid
      | Set the priority of Service_ovrdflg higher than Cal_ovrdflg
      | In this way, the Cal_ovrd can be automatically disabled in production
  signal_valid_flg_raw : Inport
  signal_raw : Inport  Port=2
  cal_ovrdflg : Inport  Port=3
  cal_ovrdval : Inport  Port=4
  Data Type Duplicate : DataTypeDuplicate  NumInputPorts=3
  Switch1 : Switch  Criteria=u2 ~= 0  Threshold=0.5
  Switch2 : Switch  Criteria=u2 ~= 0  Threshold=0.5
  True : Constant  Value=TRUE  OutDataTypeStr=boolean
  signal : Outport
  signal_valid_flg : Outport  Port=2
  wires:
  signal_valid_flg_raw/1 -> Switch2/3  "signal_valid_flg_raw"
  Switch2/1 -> signal_valid_flg/1  "signal_valid_flg"
  True/1 -> Switch2/1
  signal_raw/1 -> Switch1/3, Data Type Duplicate/1  "signal_raw"
  cal_ovrdval/1 -> Switch1/1, Data Type Duplicate/2  "cal_ovrdval"
  cal_ovrdflg/1 -> Switch1/2, [cal_ovrdflg]  "cal_ovrdflg"
  [cal_ovrdflg] -> Switch2/2
  Switch1/1 -> signal/1, Data Type Duplicate/3  "signal"

== system hcu_lib/Signal_Process_Blocks/override_signal_m2  ==
  note: When either service_ovrdflg or cal_ovrdflg is true, signal_valid_flg is set as TRUE
  note: ONLY ONE ovrdflg (Service_ovrdflg and Cal_ovrdflg) can be valid
      | Set the priority of Service_ovrdflg higher than Cal_ovrdflg
      | In this way, the Cal_ovrd can be automatically disabled in production
  signal_valid_flg_raw : Inport
  signal_raw : Inport  Port=2
  service_ovrdflg : Inport  Port=3
  service_ovrdval : Inport  Port=4
  cal_ovrdflg : Inport  Port=5
  cal_ovrdval : Inport  Port=6
  Data Type Duplicate : DataTypeDuplicate  NumInputPorts=5
  Logical Operator : Logic  Operator=OR  AllPortsSameDT=off  OutDataTypeStr=boolean
  Switch : Switch  Criteria=u2 ~= 0  Threshold=0.5
  Switch1 : Switch  Criteria=u2 ~= 0  Threshold=0.5
  Switch2 : Switch  Criteria=u2 ~= 0  Threshold=0.5
  True : Constant  Value=TRUE  OutDataTypeStr=boolean
  signal : Outport
  signal_valid_flg : Outport  Port=2
  wires:
  signal_valid_flg_raw/1 -> Switch2/3  "signal_valid_flg_raw"
  Switch2/1 -> signal_valid_flg/1  "signal_valid_flg"
  True/1 -> Switch2/1
  Logical Operator/1 -> Switch2/2
  Switch1/1 -> Switch/3, Data Type Duplicate/4
  signal_raw/1 -> Switch1/3, Data Type Duplicate/1  "signal_raw"
  cal_ovrdval/1 -> Switch1/1, Data Type Duplicate/2  "cal_ovrdval"
  service_ovrdval/1 -> Switch/1, Data Type Duplicate/3  "service_ovrdval"
  cal_ovrdflg/1 -> Switch1/2, [cal_ovrdflg]  "cal_ovrdflg"
  service_ovrdflg/1 -> Switch/2, [service_ovrdflg]  "service_ovrdflg"
  Switch/1 -> signal/1, Data Type Duplicate/5  "signal"
  [service_ovrdflg] -> Logical Operator/1
  [cal_ovrdflg] -> Logical Operator/2

== system hcu_lib/Signal_Process_Blocks/sig_valid_check ==
  new_signal : Inport
  new_signal_valid_flg : Inport  Port=2
  invalid_override : Inport  Port=3
  valid_override : Inport  Port=4
  def_value : Inport  Port=5
  sat : Inport  Port=6
  inc : Inport  Port=7
  dec : Inport  Port=8
  Logical Operator : Logic  Tag=struct('inputs','2','comment',struct('text','','placement',1),'logdata',struct('maxnumvals',inf,'plotchannels',[],'stepsize',0,'downsampling',1,'loggingmode',3,'channels',1),'operator','OR','output',struct('class','default','type','Bool8','description','','address','','unit','','name','$S_$B'),'date',731430.467498704)
  Logical Operator1 : Logic  Tag=struct('inputs','1','comment',struct('text','','placement',1),'logdata',struct('maxnumvals',inf,'plotchannels',[],'stepsize',0,'downsampling',1,'loggingmode',3,'channels',1),'operator','NOT','output',struct('class','default','type','Bool8','description','','address','','unit','','name','$S_$B'),'date',731430.46749816)  Operator=NOT  Inputs=1
  Logical Operator2 : Logic  Tag=struct('inputs','1','comment',struct('text','','placement',1),'logdata',struct('maxnumvals',inf,'plotchannels',[],'stepsize',0,'downsampling',1,'loggingmode',3,'channels',1),'operator','NOT','output',struct('class','default','type','Bool8','description','','address','','unit','','name','$S_$B'),'date',731430.46749816)  Operator=NOT  Inputs=1
  Logical Operator3 : Logic  Tag=struct('inputs','2','comment',struct('text','','placement',1),'logdata',struct('maxnumvals',inf,'plotchannels',[],'stepsize',0,'downsampling',1,'loggingmode',3,'channels',1),'operator','OR','output',struct('class','default','type','Bool8','description','','address','','unit','','name','$S_$B'),'date',731430.467498704)  Operator=OR
  Switch : Switch  Criteria=u2 ~= 0
  Switch1 : Switch  Criteria=u2 ~= 0
  Terminator : Terminator
  UnitDelay : UnitDelay  Tag=struct('comment',struct('text','','placement',1),'logdata',struct('maxnumvals',inf,'plotchannels',[],'stepsize',0,'downsampling',1,'loggingmode',3,'channels',1),'output',struct('width',1,'name','$S_$B','unit','','type','Int32Bin15','offset',0,'max',32767,'min',-32768,'freeze',1,'lsb',2^-16,'arb',0,'class','default','address','','description','','autoscalingmode',1,'lowerheadroom',1,'upperheadroom',1,'headroomunit','bit','checkmin',0,'checkmax',0,'show',0,'initial','0'),'state',0,'dt','-1','date',731401.644401968)  SampleTime=-1  HasFrameUpgradeWarning=on
  fault_filter_reset : $bdroot/Signal_Process_Blocks/fault_filter_reset
  fault_flg : Outport
  valid_signal : Outport  Port=2
  wires:
  [ifault_flg] -> fault_filter_reset/1  "ifault_flg"
  fault_filter_reset/2 -> Terminator/1  "ff_count"
  fault_filter_reset/1 -> fault_flg/1, Switch/2  "fault_flg"
  Switch/1 -> valid_signal/1, UnitDelay/1  "valid_signal"
  def_value/1 -> Switch/1  "def_value"
  Logical Operator1/1 -> Logical Operator3/1
  new_signal_valid_flg/1 -> Logical Operator1/1  "new_signal_valid_flg"
  invalid_override/1 -> Logical Operator3/2
  sat/1 -> fault_filter_reset/2  "sat"
  inc/1 -> fault_filter_reset/3  "inc"
  dec/1 -> fault_filter_reset/4  "dec"
  UnitDelay/1 -> Switch1/1  "old_signal"
  Switch1/1 -> Switch/3
  new_signal/1 -> Switch1/3  "new_signal"
  Logical Operator/1 -> [ifault_flg]  "ifault_flg"
  [ifault_flg] -> Switch1/2
  valid_override/1 -> Logical Operator2/1
  Logical Operator3/1 -> Logical Operator/1
  Logical Operator2/1 -> Logical Operator/2

== system hcu_lib/Unit_Conversion_Blocks/km2miles ==
  u : Inport
  Gain : Gain  Gain=KPH2MPH
  y : Outport
  wires:
  Gain/1 -> y/1  "y"
  u/1 -> Gain/1  "u"

== system hcu_lib/Unit_Conversion_Blocks/kph2mps ==
  u : Inport
  Gain : Gain  Gain=KPH2MPS
  y : Outport
  wires:
  Gain/1 -> y/1  "y"
  u/1 -> Gain/1  "u"

== system hcu_lib/Unit_Conversion_Blocks/kxx2xx ==
  u : Inport
  Gain : Gain  Gain=KXX2XX
  y : Outport
  wires:
  u/1 -> Gain/1  "u"
  Gain/1 -> y/1  "y"

== system hcu_lib/Unit_Conversion_Blocks/litres2gallons ==
  u : Inport
  Constant : Constant  Value=UK  OutDataTypeStr=boolean
  Switch : Switch  Threshold=0.5  ZeroCross=off
  UK : Gain  Gain=0.2199692483
  US : Gain  Gain=0.2641720524
  y : Outport
  wires:
  UK/1 -> Switch/1
  US/1 -> Switch/3
  u/1 -> UK/1, US/1  "u"
  Switch/1 -> y/1  "y"
  Constant/1 -> Switch/2

== system hcu_lib/Unit_Conversion_Blocks/miles2km ==
  u : Inport
  Gain : Gain  Gain=MPH2KPH
  y : Outport
  wires:
  u/1 -> Gain/1  "u"
  Gain/1 -> y/1  "y"

== system hcu_lib/Unit_Conversion_Blocks/mps2kph ==
  u : Inport
  Gain : Gain  Gain=MPS2KPH
  y : Outport
  wires:
  u/1 -> Gain/1  "u"
  Gain/1 -> y/1  "y"

== system hcu_lib/Unit_Conversion_Blocks/radps2rpm ==
  u : Inport
  Gain : Gain  Gain=RADPS2RPM
  y : Outport
  wires:
  u/1 -> Gain/1  "u"
  Gain/1 -> y/1  "y"

== system hcu_lib/Unit_Conversion_Blocks/rpm2radps ==
  u : Inport
  Gain : Gain  Gain=RPM2RADPS
  y : Outport
  wires:
  Gain/1 -> y/1  "y"
  u/1 -> Gain/1  "u"

== system hcu_lib/Unit_Conversion_Blocks/xx2kxx ==
  u : Inport
  Gain : Gain  Gain=XX2KXX
  y : Outport
  wires:
  u/1 -> Gain/1  "u"
  Gain/1 -> y/1  "y"

== system hcu_lib/Basic_Blocks/DIDReadData/Latch1 ==
  set : Inport
  Data Type Conversion : DataTypeConversion  OutDataTypeStr=boolean
  Switch1 : Switch  Criteria=u2 ~= 0  Threshold=0.5
      settings: AttributesFormatString=<Criteria=%<Criteria>>
  Unit Delay : UnitDelay  SampleTime=-1  HasFrameUpgradeWarning=on
  latched : Outport
  wires:
  Data Type Conversion/1 -> Switch1/2
  set/1 -> Switch1/3
  Switch1/1 -> latched/1, Unit Delay/1
  Unit Delay/1 -> Data Type Conversion/1, Switch1/1

== system hcu_lib/Basic_Blocks/DebouncedFlg/AddMinusCounter ==
  note: /* Max Value of counter is 255 */
  add_trigger : Inport
  minus_trigger : Inport  Port=2
  reset : Inport  Port=3
  max_count : Inport  Port=4
  Constant1 : Constant  Value=ZERO_INT  OutDataTypeStr=uint16
  Constant2 : Constant  Value=ONE_INT  OutDataTypeStr=uint16
  Constant3 : Constant  Value=ONE_INT  OutDataTypeStr=uint16
  MinMax : MinMax  Inputs=2
  Saturation : Saturate  UpperLimit=255  LowerLimit=0  OutDataTypeStr=uint8
      settings: AttributesFormatString=<upper = %<UpperLimit>>\n<lower = %<LowerLimit>>
  Saturation2 : Saturate  UpperLimit=255  LowerLimit=1  OutDataTypeStr=uint8
      settings: AttributesFormatString=<upper = %<UpperLimit>>\n<lower = %<LowerLimit>>
  Saturation4 : Saturate  UpperLimit=254  LowerLimit=0  OutDataTypeStr=uint8
      settings: AttributesFormatString=<upper = %<UpperLimit>>\n<lower = %<LowerLimit>>
  Subtract1 : Sum  Inputs=+-
  Subtract2 : Sum
  Switch1 : Switch  Criteria=u2 ~= 0
      settings: AttributesFormatString=<%<Criteria>>
  Switch2 : Switch  Criteria=u2 ~= 0
      settings: AttributesFormatString=<%<Criteria>>
  Switch3 : Switch  Criteria=u2 ~= 0
      settings: AttributesFormatString=<%<Criteria>>
  Unit Delay1 : UnitDelay  SampleTime=-1  HasFrameUpgradeWarning=on
      settings: AttributesFormatString=<initial = %<X0>>
  count : Outport
  wires:
  Saturation/1 -> MinMax/1
  max_count/1 -> Saturation/1
  Unit Delay1/1 -> Switch2/3, [last_count]
  MinMax/1 -> count/1, Unit Delay1/1
  Constant1/1 -> Switch1/1
  reset/1 -> Switch1/2
  add_trigger/1 -> Switch2/2
  Constant2/1 -> Subtract2/2
  Switch3/1 -> Switch1/3
  Switch2/1 -> Switch3/3
  minus_trigger/1 -> Switch3/2
  Constant3/1 -> Subtract1/2
  Switch1/1 -> MinMax/2
  [last_count] -> Saturation4/1
  Saturation4/1 -> Subtract2/1
  Subtract1/1 -> Switch3/1
  Saturation2/1 -> Subtract1/1
  [last_count] -> Saturation2/1
  Subtract2/1 -> Switch2/1

== system hcu_lib/Basic_Blocks/DebouncedFlg/SR_Latch ==
  set : Inport
  reset : Inport  Port=2
  Data Type Conversion : DataTypeConversion  OutDataTypeStr=boolean
  Logical Operator : Logic  AllPortsSameDT=off  OutDataTypeStr=boolean
  Logical Operator1 : Logic  Operator=NOT  AllPortsSameDT=off  OutDataTypeStr=boolean
  Switch1 : Switch  Criteria=u2 ~= 0  Threshold=0.5
      settings: AttributesFormatString=<Criteria=%<Criteria>>
  Switch2 : Switch  Criteria=u2 ~= 0  Threshold=0.5
      settings: AttributesFormatString=<Criteria=%<Criteria>>
  Unit Delay : UnitDelay  SampleTime=-1  HasFrameUpgradeWarning=on
  latched : Outport
  wires:
  Logical Operator1/1 -> Switch2/1, Logical Operator/2
  Logical Operator/1 -> Switch1/2
  Switch2/1 -> Switch1/3
  Unit Delay/1 -> Switch2/3
  reset/1 -> Logical Operator1/1, Switch2/2
  set/1 -> Logical Operator/1, Switch1/1
  Switch1/1 -> Data Type Conversion/1
  Data Type Conversion/1 -> latched/1, Unit Delay/1

== system hcu_lib/Basic_Blocks/DebouncedFlg/Timer ==
  note: /* output signal type is single */
  trigger : Inport
  reset : Inport  Port=2
  Ts : Inport  Port=3
  max_time : Inport  Port=4
  Constant1 : Constant  Value=ZERO_FLOAT  OutDataTypeStr=single
  GreaterThan : RelationalOperator  Operator=<=  OutDataTypeStr=boolean  RndMeth=Simplest
  Subtract2 : Sum
  Switch : Switch  Criteria=u2 > Threshold
  Switch1 : Switch  Criteria=u2 ~= 0
      settings: AttributesFormatString=<%<Criteria>>
  Switch2 : Switch  Criteria=u2 ~= 0
      settings: AttributesFormatString=<%<Criteria>>
  Unit Delay1 : UnitDelay  SampleTime=-1  HasFrameUpgradeWarning=on
      settings: AttributesFormatString=<initial = %<X0>>
  time : Outport
  wires:
  [last_time] -> Subtract2/1
  max_time/1 -> Switch/1, GreaterThan/1
  Unit Delay1/1 -> [last_time], Switch1/3
  Switch/1 -> time/1, Unit Delay1/1
  Switch2/1 -> Switch/3, GreaterThan/2
  Ts/1 -> Subtract2/2
  Switch1/1 -> Switch2/3
  Constant1/1 -> Switch1/1
  reset/1 -> Switch1/2
  trigger/1 -> Switch2/2
  Subtract2/1 -> Switch2/1
  GreaterThan/1 -> Switch/2

== system hcu_lib/Basic_Blocks/ITRI_DTC_Record/Event Status Enum ==
  Event Status Value : Constant  Value=EventStatusEnum(EventStatusIndex)  OutDataTypeStr=uint8
  Event Status : Outport
  wires:
  Event Status Value/1 -> Event Status/1

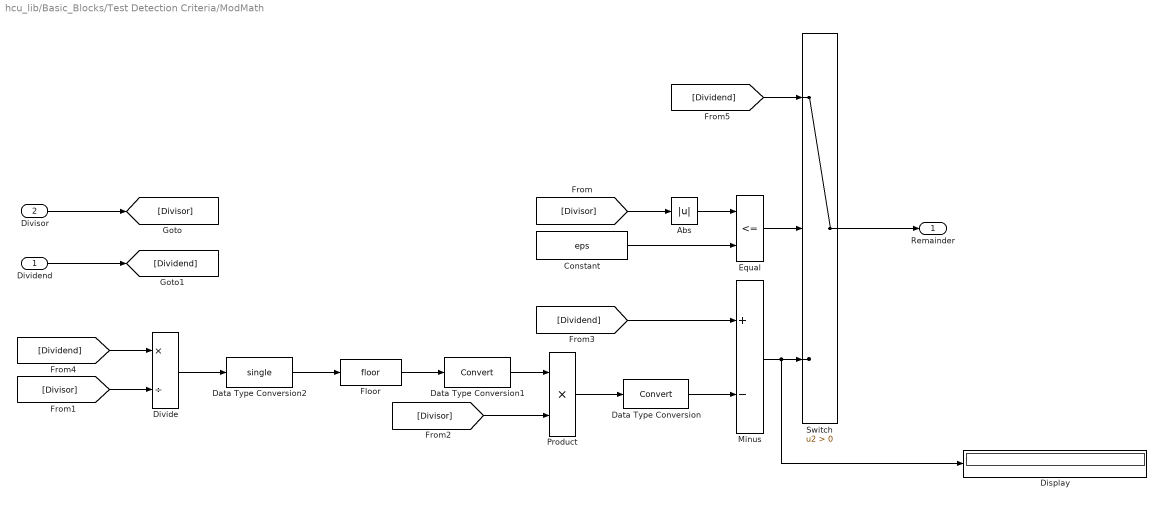
== system hcu_lib/Basic_Blocks/Test Detection Criteria/ModMath ==
  Dividend : Inport
  Divisor : Inport  Port=2
  Abs : Abs
  Constant : Constant  Value=eps
  Data Type Conversion : DataTypeConversion
  Data Type Conversion1 : DataTypeConversion
  Data Type Conversion2 : DataTypeConversion  OutDataTypeStr=single
  Display : Display
      settings: Format=long_e
  Divide : Product  Inputs=*/
  Equal : RelationalOperator  Operator=<=  OutDataTypeStr=boolean  RndMeth=Simplest
  Floor : Rounding
  Minus : Sum  Inputs=+-
  Product : Product
  Switch : Switch  Criteria=u2 > Threshold
  Remainder : Outport
  wires:
  Divisor/1 -> [Divisor]
  Equal/1 -> Switch/2
  Constant/1 -> Equal/2
  [Dividend] -> Divide/1
  Switch/1 -> Remainder/1
  [Dividend] -> Switch/1
  Minus/1 -> Display/1, Switch/3
  Data Type Conversion2/1 -> Floor/1
  Data Type Conversion/1 -> Minus/2
  [Dividend] -> Minus/1
  Dividend/1 -> [Dividend]
  Floor/1 -> Data Type Conversion1/1
  Data Type Conversion1/1 -> Product/1
  [Divisor] -> Divide/2
  Abs/1 -> Equal/1
  [Divisor] -> Product/2
  Divide/1 -> Data Type Conversion2/1
  Product/1 -> Data Type Conversion/1
  [Divisor] -> Abs/1

== system hcu_lib/Basic_Blocks/Test Detection Criteria/Timer ==
  note: /* output signal type is single */
  trigger : Inport
  reset : Inport  Port=2
  Ts : Inport  Port=3
  max_time : Inport  Port=4
  Constant1 : Constant  Value=ZERO_FLOAT  OutDataTypeStr=single
  MinMax : MinMax  Inputs=2
  Subtract2 : Sum
  Switch1 : Switch  Criteria=u2 ~= 0
      settings: AttributesFormatString=<%<Criteria>>
  Switch2 : Switch  Criteria=u2 ~= 0
      settings: AttributesFormatString=<%<Criteria>>
  Unit Delay1 : UnitDelay  SampleTime=-1  HasFrameUpgradeWarning=on
      settings: AttributesFormatString=<initial = %<X0>>
  time : Outport
  wires:
  Subtract2/1 -> Switch2/1
  trigger/1 -> Switch2/2
  reset/1 -> Switch1/2
  Constant1/1 -> Switch1/1
  Switch1/1 -> Switch2/3
  Ts/1 -> Subtract2/2
  Switch2/1 -> MinMax/2
  MinMax/1 -> time/1, Unit Delay1/1
  Unit Delay1/1 -> Switch1/3, [last_time]
  max_time/1 -> MinMax/1
  [last_time] -> Subtract2/1
